simulink library "ChangeFrame"  (R2014b)
settings: Solver=ode45  StartTime=0.0  StopTime=10.0  RelTol=1e-3
libraries: Qinverse x1
settings Model: Creator=Hp  LastModifiedBy=Hp

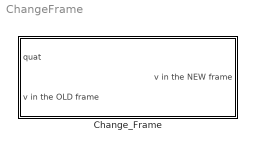
== system ChangeFrame ==
  Change_Frame : Subsystem

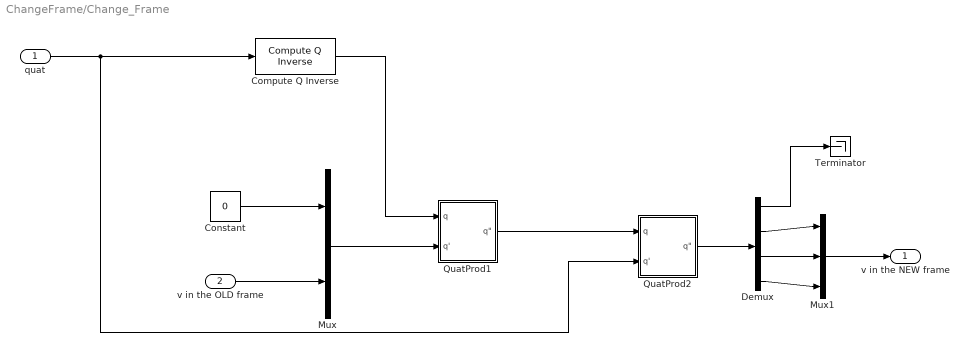
== system ChangeFrame/Change_Frame ==
  quat : Inport
  v in the OLD frame : Inport  Port=2
  Compute Q Inverse : Qinverse/Compute Q Inverse
  Constant : Constant  Value=0
  Demux : Demux
  Mux : Mux  Inputs=2
  Mux1 : Mux  Inputs=3
  QuatProd1 : Subsystem  TreatAsAtomicUnit=on
      settings: RTWFcnNameOpts=Use subsystem name  RTWFileNameOpts=Use subsystem name
  QuatProd2 : Subsystem  TreatAsAtomicUnit=on
      settings: RTWFcnNameOpts=Use subsystem name  RTWFileNameOpts=Use subsystem name
  Terminator : Terminator
  v in the NEW frame : Outport
  wires:
  quat/1 -> Compute Q Inverse/1, QuatProd2/2(q')
  Demux/1 -> Terminator/1
  v in the OLD frame/1 -> Mux/2
  Mux/1 -> QuatProd1/2(q')
  Constant/1 -> Mux/1
  Compute Q Inverse/1 -> QuatProd1/1(q)
  Mux1/1 -> v in the NEW frame/1
  Demux/2 -> Mux1/1
  Demux/3 -> Mux1/2
  Demux/4 -> Mux1/3
  QuatProd1/1("q\"") -> QuatProd2/1(q)
  QuatProd2/1("q\"") -> Demux/1

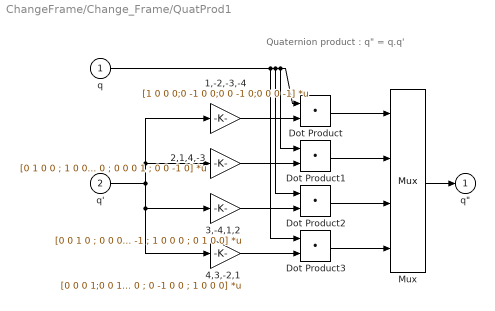
== system ChangeFrame/Change_Frame/QuatProd1 ==
  note: Quaternion product : q" = q.q'
  q : Inport  OutDataTypeStr=double  PortDimensions=4
  q' : Inport  Port=2  OutDataTypeStr=double  PortDimensions=4
  1,-2,-3,-4 : Gain  Gain=[1 0 0 0;0 -1 0 0;0 0 -1 0;0 0 0 -1]  Multiplication=Matrix(K*u) (u vector)  SaturateOnIntegerOverflow=on  OutDataTypeStr=Inherit: Same as input  ParamDataTypeStr=Inherit: Same as input
  2,1,4,-3 : Gain  Gain=[0 1 0 0 ; 1 0 0 0 ; 0 0 0 1 ; 0 0 -1 0]  Multiplication=Matrix(K*u) (u vector)  SaturateOnIntegerOverflow=on  OutDataTypeStr=Inherit: Same as input  ParamDataTypeStr=Inherit: Same as input
  3,-4,1,2 : Gain  Gain=[0 0 1 0 ; 0 0 0 -1 ; 1 0 0 0 ; 0 1 0 0]  Multiplication=Matrix(K*u) (u vector)  SaturateOnIntegerOverflow=on  OutDataTypeStr=Inherit: Same as input  ParamDataTypeStr=Inherit: Same as input
  4,3,-2,1 : Gain  Gain=[0 0 0 1;0 0 1 0 ; 0 -1 0 0 ; 1 0 0 0]  Multiplication=Matrix(K*u) (u vector)  SaturateOnIntegerOverflow=on  OutDataTypeStr=Inherit: Same as input  ParamDataTypeStr=Inherit: Same as input
  Dot Product{,1..3} (4 alike) : DotProduct  InputSameDT=on  OutDataTypeStr=Inherit: Inherit via internal rule
  Mux : Mux
  "q\"" : Outport  OutDataTypeStr=double  PortDimensions=4  InitialOutput=0
  wires:
  q'/1 -> 3,-4,1,2/1, 4,3,-2,1/1, 1,-2,-3,-4/1, 2,1,4,-3/1
  1,-2,-3,-4/1 -> Dot Product/2
  2,1,4,-3/1 -> Dot Product1/2
  3,-4,1,2/1 -> Dot Product2/2
  4,3,-2,1/1 -> Dot Product3/2
  q/1 -> Dot Product/1, Dot Product1/1, Dot Product2/1, Dot Product3/1
  Dot Product/1 -> Mux/1
  Dot Product1/1 -> Mux/2
  Dot Product2/1 -> Mux/3
  Dot Product3/1 -> Mux/4
  Mux/1 -> "q\""/1

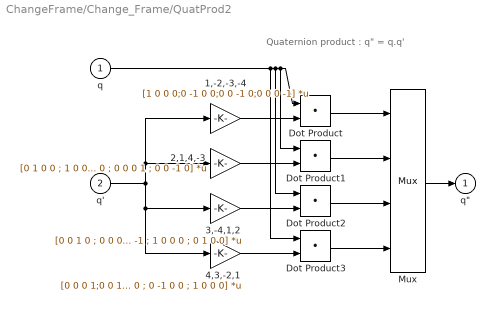
== system ChangeFrame/Change_Frame/QuatProd2 ==
  note: Quaternion product : q" = q.q'
  q : Inport  OutDataTypeStr=double  PortDimensions=4
  q' : Inport  Port=2  OutDataTypeStr=double  PortDimensions=4
  1,-2,-3,-4 : Gain  Gain=[1 0 0 0;0 -1 0 0;0 0 -1 0;0 0 0 -1]  Multiplication=Matrix(K*u) (u vector)  SaturateOnIntegerOverflow=on  OutDataTypeStr=Inherit: Same as input  ParamDataTypeStr=Inherit: Same as input
  2,1,4,-3 : Gain  Gain=[0 1 0 0 ; 1 0 0 0 ; 0 0 0 1 ; 0 0 -1 0]  Multiplication=Matrix(K*u) (u vector)  SaturateOnIntegerOverflow=on  OutDataTypeStr=Inherit: Same as input  ParamDataTypeStr=Inherit: Same as input
  3,-4,1,2 : Gain  Gain=[0 0 1 0 ; 0 0 0 -1 ; 1 0 0 0 ; 0 1 0 0]  Multiplication=Matrix(K*u) (u vector)  SaturateOnIntegerOverflow=on  OutDataTypeStr=Inherit: Same as input  ParamDataTypeStr=Inherit: Same as input
  4,3,-2,1 : Gain  Gain=[0 0 0 1;0 0 1 0 ; 0 -1 0 0 ; 1 0 0 0]  Multiplication=Matrix(K*u) (u vector)  SaturateOnIntegerOverflow=on  OutDataTypeStr=Inherit: Same as input  ParamDataTypeStr=Inherit: Same as input
  Dot Product{,1..3} (4 alike) : DotProduct  InputSameDT=on  OutDataTypeStr=Inherit: Inherit via internal rule
  Mux : Mux
  "q\"" : Outport  OutDataTypeStr=double  PortDimensions=4  InitialOutput=0
  wires:
  q'/1 -> 3,-4,1,2/1, 4,3,-2,1/1, 1,-2,-3,-4/1, 2,1,4,-3/1
  1,-2,-3,-4/1 -> Dot Product/2
  2,1,4,-3/1 -> Dot Product1/2
  3,-4,1,2/1 -> Dot Product2/2
  4,3,-2,1/1 -> Dot Product3/2
  q/1 -> Dot Product/1, Dot Product1/1, Dot Product2/1, Dot Product3/1
  Dot Product/1 -> Mux/1
  Dot Product1/1 -> Mux/2
  Dot Product2/1 -> Mux/3
  Dot Product3/1 -> Mux/4
  Mux/1 -> "q\""/1
